simulink model "mcb_pmsm_foc_sensorless_CVAC_IF_f28379d"  (R2026a)
settings: Solver=FixedStepDiscrete  StopTime=8  EnableMultiTasking=on
InitFcn:
  | cvac_if_model_init;
model workspace (MAT data in the model file):
  encoderResolution = 2000
  hallOffset = '0.5'
  indexOffset = 850
  polePairs = '4'
values from neighbouring files (symbols this model uses):
  acceleration = 500 / PU_System.N_base    [cvac_if_model_init.m]
  CVAC_IF_Mode = uint8(2)    [cvac_if_model_init.m]
  CVAC_LoadConstant = CVAC_LoadFinal    [cvac_if_model_init.m]
  PU_System = mcb.getPUSystemParameters(pmsm, inverter)    [cvac_if_model_init.m]
  Speed_openLoop_PU = 400 / PU_System.N_base    [cvac_if_model_init.m]
  Ts = single(param.TsFast)    [cvac_if_reference_fast_step.m]
undefined symbols (not defined in the file or in its folder): bit, CVAC_LoadFinal, CVAC_LoadInitial, CVAC_LoadStepTime, dataType, Down, GPTRIP1SEL, GPTRIP2SEL, inverter, NumBits1, NumBits2, PI_params, pmsm, Slope1, Slope2, target, Ts_motor, Ts_simulink, Ts_speed, TZ1, TZ2, Up
libraries: mcbcontrolslib x9, c2802xlib x7, simulink x6, c280xlib x5, mcbeeMathTransformLib x4, c2837xDlib x4, mcbpositiondecoderlib x3, slpidlib x3, sl_signal_attributes x2, mcbpmsmiflib x2, mcbsensorlessestimatorlib x1, svdschedulerlib x1
(part 1 of 3)
Description:
  | MIL-only CVAC I-f study model using a 540 V paper IPMSM. Do not Build or Deploy.
settings Model: ExtModeTrigDuration=8  Creator=The MathWorks, Inc.  LastModifiedBy=ASUS
settings OptimizationCC: DefaultUnderspecifiedDataType=single  OptimizeBlockIOStorage=off  BufferReuse=off  GlobalBufferReuse=off  ExpressionFolding=off  LocalBlockOutputs=off  InitFltsAndDblsToZero=on  NoFixptDivByZeroProtection=on  EfficientFloat2IntCast=on  EfficientMapNaN2IntZero=off  LifeSpan=Inf  MaxStackSize=1024  OptimizeDataStoreBuffers=off  BusAssignmentInplaceUpdate=off  DenormalBehavior=FlushToZero
settings DebuggingCC: ReadBeforeWriteMsg=DisableAll  WriteAfterWriteMsg=DisableAll  WriteAfterReadMsg=DisableAll  CheckSSInitialOutputMsg=off  InheritedTsInSrcMsg=none  MultiTaskDSMMsg=none  MultiTaskCondExecSysMsg=none  TasksWithSamePriorityMsg=none  SigSpecEnsureSampleTimeMsg=none  IntegerOverflowMsg=none  ParameterPrecisionLossMsg=none  SubsystemReferenceDiagnosticForUnitTest=warning  IntegerSaturationMsg=none
settings HardwareCC: ProdBitPerChar=16.0  ProdBitPerInt=16.0  ProdLargestAtomicInteger=Integer  ProdWordSize=16.0  ProdHWDeviceType=Texas Instruments->C2000  TargetBitPerChar=16.0  TargetBitPerInt=16.0  TargetBitPerPointer=16.0  TargetLargestAtomicInteger=Integer  TargetIntDivRoundTo=Zero  TargetEndianess=LittleEndian  TargetWordSize=16.0  TargetHWDeviceType=TI C2000
settings RTWCC: SystemTargetFile=ert.tlc  HardwareBoard=TI Delfino F28379D LaunchPad  PostCodeGenCommand=error('CVAC_IF_sim:MilOnly', 'MIL-only 540 V paper model: Build and Deploy are intentionally disabled.')  GenerateReport=on  Toolchain=Texas Instruments Code Composer Studio (C2000)  IncludeHyperlinkInReport=on  LaunchReport=on  GenerateTraceInfo=on  GenerateTraceReport=on  GenerateTraceReportSl=on  GenerateTraceReportSf=on  GenerateTraceReportEml=on  Description=Embedded Coder
settings CodeAppCC: CustomSymbolStrType=$N$R$M  InternalIdentifier=Classic
settings ERTTargetCC: ExtModeStaticAllocSize=10000.0  MemSecPackage=tic2000demospkg  CodeReplacementLibrary=TI C28x  MultiwordLength=2048.0
settings SimscapeCC: SimscapeNominalValues="[{\"value\":\"1\",\"unit\":\"A\"},{\"value\":\"1\",\"unit\":\"bar\"},{\"value\":\"1\",\"unit\":\"cm^2\"},{\"value\":\"1\",\"unit\":\"cm^3/s\"},{\"value\":\"1\",\"unit\":\"kJ/kg\"},{\"value\":\"1\",\"unit\":\"kW\"},{\"value\":\"1\",\"unit\":\"l\"},{\"value\":\"1\",\"unit\":\"N\"},{\"value\":\"1\",\"unit\":\"N*m\"},{\"value\":\"1\",\"unit\":\"V\"}]"  SimscapeLogType=none  SimscapeLogDataHistory=5000.0

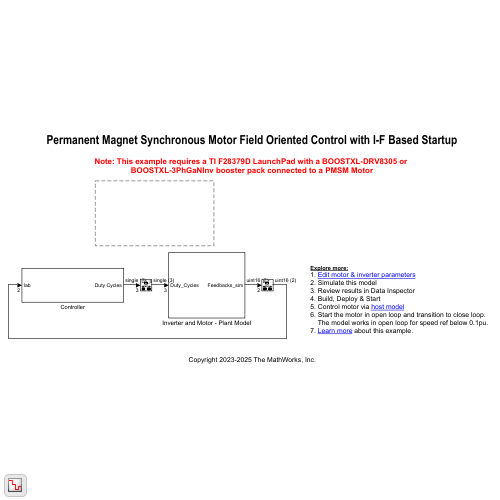
[thumbnail: Simulink's stored preview of the top-level diagram]
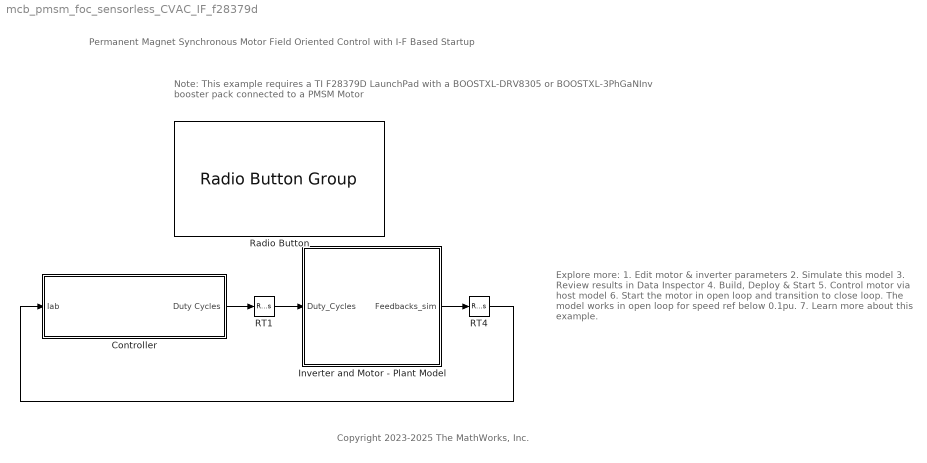
== system mcb_pmsm_foc_sensorless_CVAC_IF_f28379d ==
  note: Permanent Magnet Synchronous Motor Field Oriented Control with I-F Based Startup
  note: Explore more:
      | 1. Edit motor & inverter parameters
      | 2. Simulate this model
      | 3. Review results in Data Inspector
      | 4. Build, Deploy & Start
      | 5. Control motor via host model
      | 6. Start the motor in open loop and transition to close loop.
      | The model works in open loop for speed ref below 0.1pu.
      | 7. Learn more about this example.
  note: Note: This example requires a TI F28379D LaunchPad with a BOOSTXL-DRV8305 or
      | BOOSTXL-3PhGaNInv booster pack connected to a PMSM Motor
  note: Copyright 2023-2025 The MathWorks, Inc.
  Controller : Subsystem
  Inverter and Motor - Plant Model : Subsystem
  RT1 : RateTransition  Deterministic=off
  RT4 : RateTransition  Deterministic=off
  Radio Button : RadioButtonGroup  LabelPosition=Hide  SelectedLabel=Extended Emf observer  ButtonGroupName=Postion Estimator
  wires:
  Inverter and Motor - Plant Model/1(Feedbacks_sim) -> RT4/1
  RT1/1 -> Inverter and Motor - Plant Model/1(Duty_Cycles)
  RT4/1 -> Controller/1(Iab)
  Controller/1(Duty Cycles) -> RT1/1

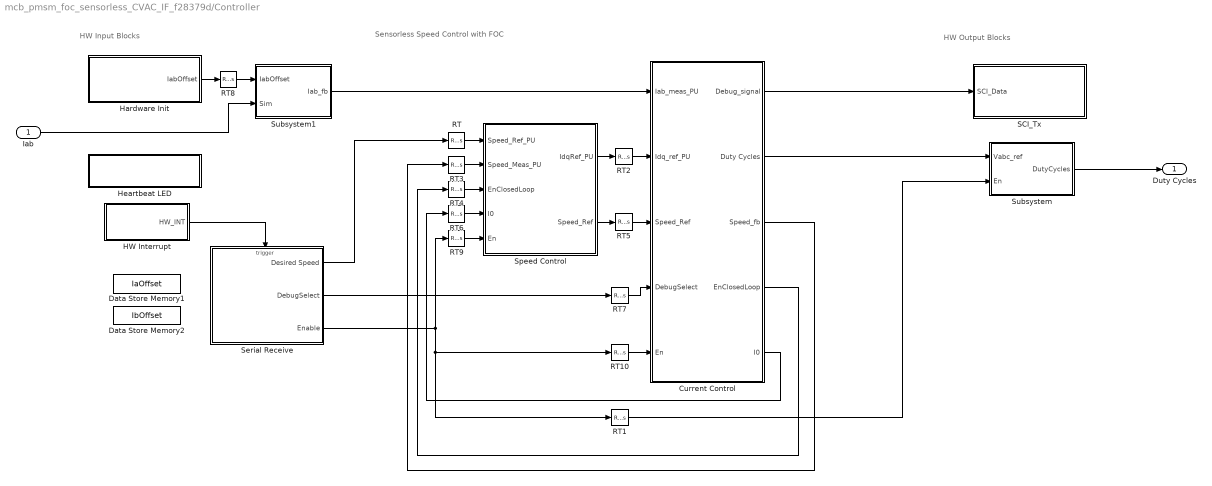
== system mcb_pmsm_foc_sensorless_CVAC_IF_f28379d/Controller ==
  note: HW Input Blocks
  note: Sensorless Speed Control with FOC
  note: HW Output Blocks
  Iab : Inport
  Current Control : Subsystem
  Data Store Memory1 : DataStoreMemory  DataStoreName=IaOffset  InitialValue=inverter.CtSensAOffset  ShowAdditionalParam=off  OutDataTypeStr=uint16
  Data Store Memory2 : DataStoreMemory  DataStoreName=IbOffset  InitialValue=inverter.CtSensBOffset  ShowAdditionalParam=off
  HW Interrupt : Subsystem  Variant=on  VariantControlMode=sim codegen switching
  Hardware Init : Subsystem  TreatAsAtomicUnit=on
  Heartbeat LED : Subsystem  TreatAsAtomicUnit=on
  RT{,3..4,6,9} (5 alike) : RateTransition  Deterministic=off  OutPortSampleTime=Ts_speed
  RT{1..2,5,7..8,10} (6 alike) : RateTransition  Deterministic=off  OutPortSampleTime=Ts
  SCI_Tx : Subsystem  Variant=on  VariantControlMode=sim codegen switching
  Serial Receive : Subsystem  SystemSampleTime=1e-3
  Speed Control : Subsystem  TreatAsAtomicUnit=on  SystemSampleTime=Ts_speed
  Subsystem : Subsystem
  Subsystem1 : Subsystem
  Duty Cycles : Outport
  wires:
  Speed Control/1(IdqRef_PU) -> RT2/1
  RT5/1 -> Current Control/3(Speed_Ref)
  RT/1 -> Speed Control/1(Speed_Ref_PU)
  Current Control/3(Speed_fb) -> RT3/1
  Speed Control/2(Speed_Ref) -> RT5/1
  RT2/1 -> Current Control/2(Idq_ref_PU)
  RT3/1 -> Speed Control/2(Speed_Meas_PU)
  Serial Receive/1(Desired Speed) -> RT/1
  Iab/1 -> Subsystem1/2(Sim)
  HW Interrupt/1(HW_INT) -> Serial Receive/Trigger
  Current Control/1(Debug_signal) -> SCI_Tx/1(SCI_Data)
  Subsystem/1(DutyCycles) -> Duty Cycles/1
  Current Control/2(Duty Cycles) -> Subsystem/1(Vabc_ref)
  Serial Receive/3(Enable) -> RT1/1, RT10/1, RT9/1
  RT10/1 -> Current Control/5(En)
  RT1/1 -> Subsystem/2(En)
  Current Control/4(EnClosedLoop) -> RT4/1
  Current Control/5(I0) -> RT6/1
  RT4/1 -> Speed Control/3(EnClosedLoop)
  RT6/1 -> Speed Control/4(I0)
  Serial Receive/2(DebugSelect) -> RT7/1
  RT7/1 -> Current Control/4(DebugSelect)
  Hardware Init/1(IabOffset) -> RT8/1
  RT8/1 -> Subsystem1/1(IabOffset)
  RT9/1 -> Speed Control/5(En)
  Subsystem1/1(Iab_fb) -> Current Control/1(Iab_meas_PU)

== system mcb_pmsm_foc_sensorless_CVAC_IF_f28379d/Inverter and Motor - Plant Model ==
  Duty_Cycles : Inport
  Codegeneration : Subsystem
  Simulation : Subsystem
  Variant Sink : VariantSink  VariantControlMode=sim codegen switching  VariantControls={(codegen), (sim)}
  Variant Source1 : VariantSource  VariantControlMode=sim codegen switching  VariantControls={(codegen), (sim)}
  Feedbacks_sim : Outport  VectorParamsAs1DForOutWhenUnconnected=off
  wires:
  Duty_Cycles/1 -> Variant Sink/1
  Simulation/1(Feedbacks) -> Variant Source1/2
  Variant Sink/2 -> Simulation/1(Duty_Cycles)
  Variant Source1/1 -> Feedbacks_sim/1
  Variant Sink/1 -> Codegeneration/1(Duty_Cycles)
  Codegeneration/1(Feedbacks) -> Variant Source1/1

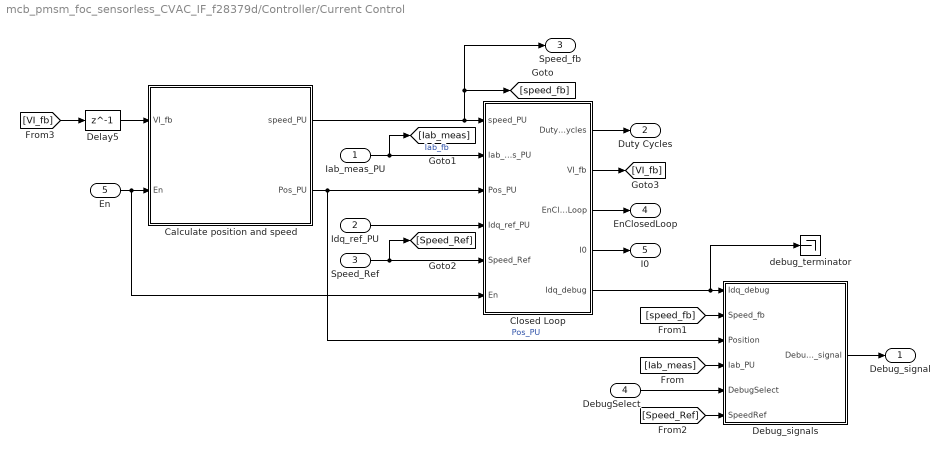
== system mcb_pmsm_foc_sensorless_CVAC_IF_f28379d/Controller/Current Control ==
  Iab_meas_PU : Inport
  Idq_ref_PU : Inport  Port=2
  Speed_Ref : Inport  Port=3
  DebugSelect : Inport  Port=4
  En : Inport  Port=5
  Calculate position and speed : Subsystem
  Closed Loop : Subsystem
  Debug_signals : Subsystem
  Delay5 : Delay  DelayLength=1
  debug_terminator : Terminator
  Debug_signal : Outport
  Duty Cycles : Outport  Port=2  InitialOutput=0  VectorParamsAs1DForOutWhenUnconnected=off
  Speed_fb : Outport  Port=3  InitialOutput=0  VectorParamsAs1DForOutWhenUnconnected=off
  EnClosedLoop : Outport  Port=4
  I0 : Outport  Port=5
  wires:
  Closed Loop/1(Duty Cycles) -> Duty Cycles/1
  Calculate position and speed/2(Pos_PU) -> Closed Loop/3(Pos_PU), Debug_signals/3(Position)  "Pos_PU"
  Idq_ref_PU/1 -> Closed Loop/4(Idq_ref_PU)
  Iab_meas_PU/1 -> Closed Loop/2(Iab_meas_PU), [Iab_meas]  "Iab_fb"
  Closed Loop/2(VI_fb) -> [VI_fb]
  [VI_fb] -> Delay5/1
  Calculate position and speed/1(speed_PU) -> Closed Loop/1(speed_PU), [speed_fb], Speed_fb/1
  Closed Loop/5(Idq_debug) -> debug_terminator/1, Debug_signals/1(Idq_debug)
  [speed_fb] -> Debug_signals/2(Speed_fb)
  Debug_signals/1(Debug_signal) -> Debug_signal/1
  Delay5/1 -> Calculate position and speed/1(VI_fb)
  En/1 -> Closed Loop/6(En), Calculate position and speed/2(En)
  DebugSelect/1 -> Debug_signals/5(DebugSelect)
  Speed_Ref/1 -> Closed Loop/5(Speed_Ref), [Speed_Ref]
  Closed Loop/3(EnClosedLoop) -> EnClosedLoop/1
  Closed Loop/4(I0) -> I0/1
  [Iab_meas] -> Debug_signals/4(Iab_PU)
  [Speed_Ref] -> Debug_signals/6(SpeedRef)

== system mcb_pmsm_foc_sensorless_CVAC_IF_f28379d/Controller/HW Interrupt ==
  Code generation : Subsystem  VariantControl=(codegen)
  Simulation : Subsystem  VariantControl=(sim)
  HW_INT : Outport  OutputFunctionCall=on

== system mcb_pmsm_foc_sensorless_CVAC_IF_f28379d/Controller/Hardware Init ==
  6PWM_Mode : Constant  Priority=1000  Value=0x3A16  OutDataTypeStr=uint16  SampleTime=-1
  ADC_Gain_Setting : Constant  Priority=1000  Value=inverter.SPI_Gain_Setting  OutDataTypeStr=uint16  SampleTime=-1
  Data Store Read1 : DataStoreRead  DataStoreName=IaOffset  IndexOptions=Index vector (dialog)  Indices=1  OutputSizes=1
  Data Store Read2 : DataStoreRead  DataStoreName=IbOffset  IndexOptions=Index vector (dialog)  Indices=1  OutputSizes=1
  Event Listener : EventListener  DisableCoverage=on  EventName=reset
  Mux : Mux  Inputs=2
  Mux1 : Mux  Inputs=2
  Variant Subsystem : Subsystem  Variant=on  VariantControlMode=sim codegen switching
  IabOffset : Outport
  wires:
  6PWM_Mode/1 -> Mux/1
  ADC_Gain_Setting/1 -> Mux/2
  Mux/1 -> Variant Subsystem/1(In1)
  Mux1/1 -> IabOffset/1
  Data Store Read1/1 -> Mux1/1
  Data Store Read2/1 -> Mux1/2

== system mcb_pmsm_foc_sensorless_CVAC_IF_f28379d/Controller/Heartbeat LED ==
  note: Heartbeat LED 1 Hz
  Heartbeat LED : Subsystem  Variant=on  VariantControlMode=sim codegen switching
  RED_LED : Constant  OutDataTypeStr=uint16  SampleTime=0.5
  wires:
  RED_LED/1 -> Heartbeat LED/1(In1)

== system mcb_pmsm_foc_sensorless_CVAC_IF_f28379d/Controller/SCI_Tx ==
  SCI_Data : Inport
  Code Generation : Subsystem  VariantControl=(codegen)
  Simulation : Subsystem  VariantControl=(sim)

== system mcb_pmsm_foc_sensorless_CVAC_IF_f28379d/Controller/Serial Receive ==
  SCI_Rx_INT : TriggerPort  TriggerType=function-call  VariantControl=Variant
  AND : Logic  IconShape=distinctive  AllPortsSameDT=off  OutDataTypeStr=boolean
  Compare To Zero : simulink/Logic and Bit Operations/Compare To Zero  relop=~=  OutDataTypeStr=boolean
  Data_Conditioning_Rx : Subsystem  Variant=on
  SCI_Rx : Subsystem  Variant=on  VariantControlMode=sim codegen switching
  unParse : Subsystem
  Desired Speed : Outport  VectorParamsAs1DForOutWhenUnconnected=off
  DebugSelect : Outport  Port=2
  Enable : Outport  Port=3  VectorParamsAs1DForOutWhenUnconnected=off
  wires:
  unParse/2(Debug_signals) -> DebugSelect/1
  unParse/1(Enable_PWM) -> AND/2
  Data_Conditioning_Rx/2(Out2) -> unParse/1(Data)
  SCI_Rx/1(Data) -> Data_Conditioning_Rx/1(In1)
  Data_Conditioning_Rx/1(Desired Speed) -> Compare To Zero/1, Desired Speed/1
  Compare To Zero/1 -> AND/1
  AND/1 -> Enable/1

== system mcb_pmsm_foc_sensorless_CVAC_IF_f28379d/Controller/Speed Control ==
  Speed_Ref_PU : Inport
  Speed_Meas_PU : Inport  Port=2
  EnClosedLoop : Inport  Port=3
  I0 : Inport  Port=4
  En : Inport  Port=5
  Constant2 : Constant  Value=0  OutDataTypeStr=dataType
  Mux : Mux  Inputs=2
  PI_Controller_Speed : Subsystem
  SlewRate1 : Subsystem
  Switch : Switch  Criteria=u2 > Threshold  SaturateOnIntegerOverflow=off  InputSameDT=off
  IdqRef_PU : Outport  VectorParamsAs1DForOutWhenUnconnected=off
  Speed_Ref : Outport  Port=2  VectorParamsAs1DForOutWhenUnconnected=off
  wires:
  Speed_Meas_PU/1 -> PI_Controller_Speed/2(N_fb)  "Speed_fb"
  Mux/1 -> IdqRef_PU/1
  Constant2/1 -> Mux/1
  PI_Controller_Speed/1(Iq_ref) -> Mux/2
  Switch/1 -> Speed_Ref/1, PI_Controller_Speed/1(N_ref)
  EnClosedLoop/1 -> PI_Controller_Speed/3(EnClosedLoop), Switch/2, SlewRate1/2(EnClosedLoop)
  SlewRate1/1(N_ref) -> Switch/1  "Speed_ref"
  Speed_Ref_PU/1 -> SlewRate1/1(Speed_Ref), Switch/3  "Speed_ref"
  I0/1 -> PI_Controller_Speed/4(I0)
  En/1 -> PI_Controller_Speed/5(En)

== system mcb_pmsm_foc_sensorless_CVAC_IF_f28379d/Controller/Subsystem ==
  Vabc_ref : Inport
  En : Inport  Port=2
  Inverter : Subsystem  Variant=on  VariantControlMode=sim codegen switching
  Mux : Mux  Inputs=2
  Output Scaling : Subsystem
  DutyCycles : Outport
  wires:
  Output Scaling/1(PWM_Duty_Cycles) -> Mux/1
  Mux/1 -> Inverter/1(Inverter Signals)
  Output Scaling/2(PWM_Enable) -> Mux/2
  Inverter/1(DutyCycles) -> DutyCycles/1
  En/1 -> Output Scaling/2(En)
  Vabc_ref/1 -> Output Scaling/1(Vabc_ref)

== system mcb_pmsm_foc_sensorless_CVAC_IF_f28379d/Controller/Subsystem1 ==
  IabOffset : Inport
  Sim : Inport  Port=2
  Calculate Phase Currents : Subsystem
  HW_Inputs : Subsystem  Variant=on  VariantControlMode=sim codegen switching
  Iab_fb : Outport
  wires:
  HW_Inputs/1(Iab_ADC) -> Calculate Phase Currents/2(Iab_ADC)
  IabOffset/1 -> Calculate Phase Currents/1(IabOffset)
  Calculate Phase Currents/1(Iab_meas_PU) -> Iab_fb/1  "Iab_fb"
  Sim/1 -> HW_Inputs/1(Sim)

== system mcb_pmsm_foc_sensorless_CVAC_IF_f28379d/Inverter and Motor - Plant Model/Codegeneration ==
  Duty_Cycles : Inport
  Ground : Ground
  Terminator : Terminator
  Feedbacks : Outport  VectorParamsAs1DForOutWhenUnconnected=off
  wires:
  Duty_Cycles/1 -> Terminator/1
  Ground/1 -> Feedbacks/1

== system mcb_pmsm_foc_sensorless_CVAC_IF_f28379d/Inverter and Motor - Plant Model/Simulation ==
  Duty_Cycles : Inport
  Bus Selector : BusSelector  OutputSignals=MtrPos
  Gain : Gain  Gain=1/(2*pi)  OutDataTypeStr=Inherit: Same as input
  Interior_PMSM_Paper : autolibpmsminterior/Interior PMSM  port_config=Torque  sim_type=Discrete  Ts=Ts_motor  P=pmsm.p  Rs=pmsm.Rs  Ldq=[pmsm.Ld,pmsm.Lq]  KConstText=Permanent flux linkage constant (lambda_pm):  lambda_pm=pmsm.FluxPM  Ke=159.9771  mechanical=[pmsm.J,pmsm.B,0]  idq0=[0 0]  theta_init=0  omega_init=0  KConst=pmsm.FluxPM  lambda_pm_calc=0.2205  Kt=0.07  RefBlkName='autolibpmsminterior/Interior PMSM'  aMode=1
  Inverter : Subsystem
  Load_Profile (Torque) : Subsystem
  Mechanical to Electrical Position : mcbpositiondecoderlib/Mechanical to Electrical Position  PolePairsInputType=Specify via dialog  NrPP=pmsm.p  selectedRange=Radians  MechOfstInputType=Specify via dialog  mechOffsetIn=0  maxAngleIn=2*pi  InputDataType=single  VariantSelect=floating-point
  RT1 : RateTransition  Deterministic=off  OutPortSampleTime=Ts_simulink
  Rate Transition : RateTransition  Deterministic=off  OutPortSampleTime=Ts_motor
  Rate Transition1 : RateTransition  Deterministic=off  OutPortSampleTime=Ts_motor
  Sensor_Measurements : Subsystem
  Terminator : Terminator
  Terminator1 : Terminator
  Feedbacks : Outport  VectorParamsAs1DForOutWhenUnconnected=off
  wires:
  Mechanical to Electrical Position/1 -> Gain/1  "MtrPosElec"
  Duty_Cycles/1 -> Inverter/1(Duty_abc)
  RT1/1 -> Sensor_Measurements/1(PhaseCurr)
  Load_Profile (Torque)/1(Load_Trq) -> Rate Transition1/1
  Inverter/1(Vabc) -> Rate Transition/1
  Bus Selector/1 -> Mechanical to Electrical Position/1  "<MtrPos>"
  Gain/1 -> Terminator1/1  "MtrPosElec"
  Sensor_Measurements/1(Sim_fb) -> Feedbacks/1
  Rate Transition1/1 -> Interior_PMSM_Paper/1
  Rate Transition/1 -> Interior_PMSM_Paper/2
  Interior_PMSM_Paper/1 -> Bus Selector/1
  Interior_PMSM_Paper/2 -> RT1/1  "Iabc"
  Interior_PMSM_Paper/3 -> Terminator/1  "MtrSpdTrue"

== system mcb_pmsm_foc_sensorless_CVAC_IF_f28379d/Controller/Current Control/Calculate position and speed ==
  VI_fb : Inport
  En : Inport  Port=2
  Demux : Demux  Outputs=2
  EstimatorSelector : Constant  OutDataTypeStr=uint32
  Extended EMF Observer : Subsystem
  Flux Observer : Subsystem
  Merge : Merge
  Switch Case : SwitchCase  CaseConditions={0,1}  ShowDefaultCase=off
  speed_PU : Outport
  Pos_PU : Outport  Port=2
  wires:
  Demux/1 -> Pos_PU/1
  Demux/2 -> speed_PU/1
  EstimatorSelector/1 -> Switch Case/1
  Flux Observer/1(Position/Speed) -> Merge/1
  Merge/1 -> Demux/1
  VI_fb/1 -> Extended EMF Observer/1(InputSignals), Flux Observer/1(InputSignals)
  Extended EMF Observer/1(Position/Speed) -> Merge/2
  Switch Case/2 -> Extended EMF Observer/Action
  Switch Case/1 -> Flux Observer/Action
  En/1 -> Extended EMF Observer/2(En), Flux Observer/2(En)

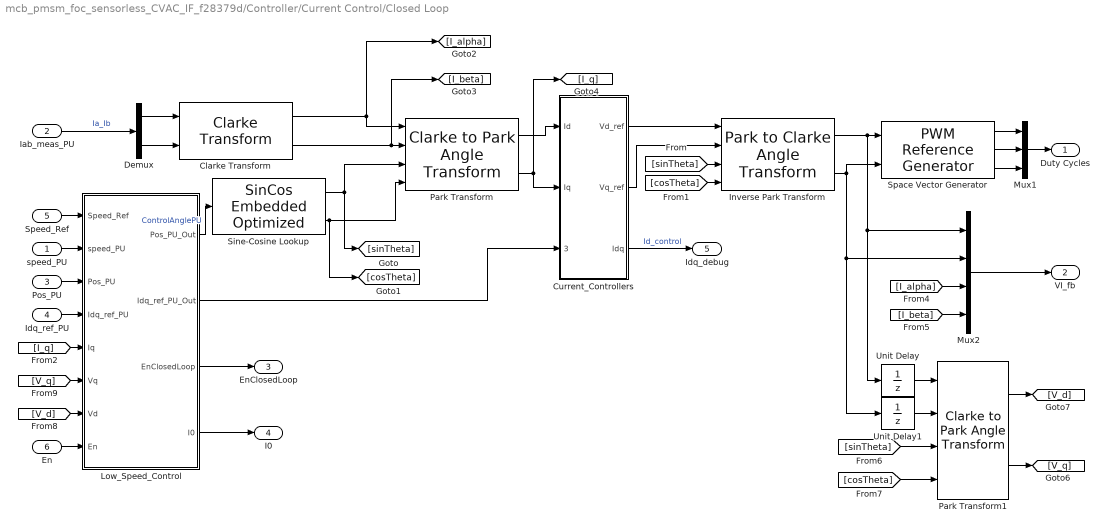
== system mcb_pmsm_foc_sensorless_CVAC_IF_f28379d/Controller/Current Control/Closed Loop ==
  speed_PU : Inport
  Iab_meas_PU : Inport  Port=2
  Pos_PU : Inport  Port=3
  Idq_ref_PU : Inport  Port=4
  Speed_Ref : Inport  Port=5
  En : Inport  Port=6
  Clarke Transform : mcbeeMathTransformLib/Clarke Transform  VariantControl=Variant2  PowerInvariant=off  UseWithEmbedded=on  PhaseInput=Two inputs
      settings: LibrarySourceBlock=mcbcontrolslib/Clarke Transform
  Current_Controllers : Subsystem
  Demux : Demux  Outputs=2
  Inverse Park Transform : mcbeeMathTransformLib/Park to Clarke Angle Transform  AxisAlignment=D-axis  UseWithEmbedded=on  PhaseInput=Two inputs  ThetaInput=Sine and Cosine electrical position  AngleInput=Per-unit  N_points=1024
      settings: LibrarySourceBlock=mcbcontrolslib/Inverse Park Transform
  Low_Speed_Control : Subsystem
  Mux1 : Mux  Inputs=3
  Mux2 : Mux
  Park Transform : mcbeeMathTransformLib/Clarke to Park Angle Transform  AxisAlignment=D-axis  UseWithEmbedded=on  PhaseInput=Two inputs  ThetaInput=Sine and Cosine electrical position  AngleInput=Per-unit  N_points=1024
      settings: LibrarySourceBlock=mcbcontrolslib/Park Transform
  Park Transform1 : mcbeeMathTransformLib/Clarke to Park Angle Transform  AxisAlignment=D-axis  UseWithEmbedded=on  PhaseInput=Two inputs  ThetaInput=Sine and Cosine electrical position  AngleInput=Per-unit  N_points=1024
      settings: LibrarySourceBlock=mcbcontrolslib/Park Transform
  Sine-Cosine Lookup : mcbcontrolslib/SinCos Embedded Optimized  LabelModeActiveChoice=MCB_Sin  OptforProc=off  OptLevelPop=Disabled  ApproximationMethod=None  UserApproxMethod=Lookup  ApproxStatus=None  ThetaDataType=single  CopyThetaDataType=single  InterpMethod=Linear point-slope  NumberOfDataPoints=16  NumberOfIterations=11  RemoveProtectionAgainstOutOfRangeInput=off  TableDataTypeStr=Inherit: Inherit via input  AngleInput=Per-unit  CopyAngleInput=Per-unit  N_points=1024  CopyN_points=1024  Datatype=single  CopyTableDatatype=single  DatatypeInput=Inherit from input  IsPrevStrictOpt=0  IsPrevLUTForced=0
  Space Vector Generator : mcbcontrolslib/PWM Reference Generator  modType=SVM: space vector modulation  inSignal=Valphabeta  expandVoltageInput=on  inputUnits=Per-unit  LimitModulation=off  enableVoltage=on  enableModulationSignal=off  enableDutyCycle=off  expandVoltageOutput=on
  Unit Delay : UnitDelay  SampleTime=-1
  Unit Delay1 : UnitDelay  SampleTime=-1
  Duty Cycles : Outport  VectorParamsAs1DForOutWhenUnconnected=off
  VI_fb : Outport  Port=2  VectorParamsAs1DForOutWhenUnconnected=off
  EnClosedLoop : Outport  Port=3
  I0 : Outport  Port=4
  Idq_debug : Outport  Port=5  VectorParamsAs1DForOutWhenUnconnected=off
  wires:
  Current_Controllers/1(Vd_ref) -> Inverse Park Transform/1
  [cosTheta] -> Inverse Park Transform/4
  [I_beta] -> Mux2/4
  Inverse Park Transform/2 -> Mux2/2, Unit Delay1/1, Space Vector Generator/2
  Inverse Park Transform/1 -> Mux2/1, Unit Delay/1, Space Vector Generator/1
  [sinTheta] -> Inverse Park Transform/3
  Mux2/1 -> VI_fb/1
  Clarke Transform/1 -> Park Transform/1, [I_alpha]
  Current_Controllers/2(Vq_ref) -> Inverse Park Transform/2
  Clarke Transform/2 -> [I_beta], Park Transform/2
  Sine-Cosine Lookup/1 -> Park Transform/3, [sinTheta]
  [I_alpha] -> Mux2/3
  Space Vector Generator/1 -> Mux1/1
  Space Vector Generator/3 -> Mux1/3
  Mux1/1 -> Duty Cycles/1
  Sine-Cosine Lookup/2 -> Park Transform/4, [cosTheta]
  Space Vector Generator/2 -> Mux1/2
  Park Transform/1 -> Current_Controllers/1(Id)
  Park Transform/2 -> Current_Controllers/2(Iq), [I_q]
  Demux/1 -> Clarke Transform/1
  Demux/2 -> Clarke Transform/2
  Iab_meas_PU/1 -> Demux/1  "Ia_Ib"
  Pos_PU/1 -> Low_Speed_Control/3(Pos_PU)
  Current_Controllers/3(Idq) -> Idq_debug/1  "Id_control"
  Low_Speed_Control/1(Pos_PU_Out) -> Sine-Cosine Lookup/1  "ControlAnglePU"
  speed_PU/1 -> Low_Speed_Control/2(speed_PU)
  Idq_ref_PU/1 -> Low_Speed_Control/4(Idq_ref_PU)
  [I_q] -> Low_Speed_Control/5(Iq)
  Low_Speed_Control/2(Idq_ref_PU_Out) -> Current_Controllers/3(Idq_Ref)
  Speed_Ref/1 -> Low_Speed_Control/1(Speed_Ref)
  Unit Delay/1 -> Park Transform1/1
  Unit Delay1/1 -> Park Transform1/2
  [sinTheta] -> Park Transform1/3
  [cosTheta] -> Park Transform1/4
  Park Transform1/1 -> [V_d]
  Park Transform1/2 -> [V_q]
  [V_d] -> Low_Speed_Control/7(Vd)
  [V_q] -> Low_Speed_Control/6(Vq)
  En/1 -> Low_Speed_Control/8(En)
  Low_Speed_Control/3(EnClosedLoop) -> EnClosedLoop/1
  Low_Speed_Control/4(I0) -> I0/1

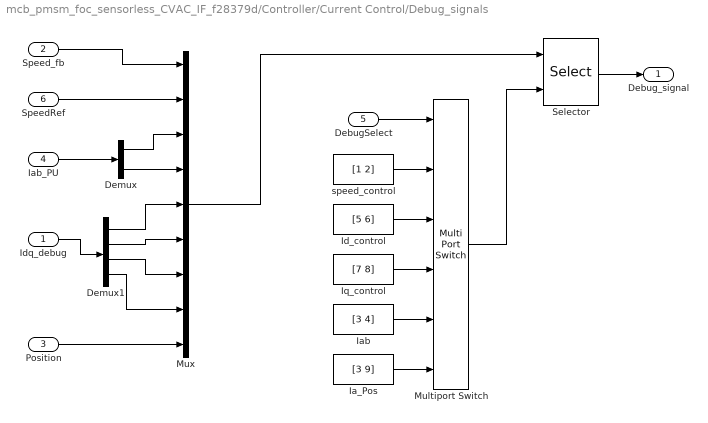
== system mcb_pmsm_foc_sensorless_CVAC_IF_f28379d/Controller/Current Control/Debug_signals ==
  Idq_debug : Inport
  Speed_fb : Inport  Port=2
  Position : Inport  Port=3
  Iab_PU : Inport  Port=4
  DebugSelect : Inport  Port=5
  SpeedRef : Inport  Port=6
  Demux : Demux  Outputs=2
  Demux1 : Demux
  Ia_Pos : Constant  Value=[3 9]  OutDataTypeStr=uint16  SampleTime=-1
  Iab : Constant  Value=[3 4]  OutDataTypeStr=uint16  SampleTime=-1
  Id_control : Constant  Value=[5 6]  OutDataTypeStr=uint16  SampleTime=-1
  Iq_control : Constant  Value=[7 8]  OutDataTypeStr=uint16  SampleTime=-1
  Multiport Switch : MultiPortSwitch  Inputs=5  DiagnosticForDefault=Warning  OutDataTypeStr=uint16  RndMeth=Simplest  SaturateOnIntegerOverflow=off  InputSameDT=off
  Mux : Mux  Inputs=9
  Selector : Selector  InputPortWidth=9  IndexOptions=Index vector (port)  Indices=[1 3]  OutputSizes=1
  speed_control : Constant  Value=[1 2]  OutDataTypeStr=uint16  SampleTime=-1
  Debug_signal : Outport
  wires:
  speed_control/1 -> Multiport Switch/2
  Id_control/1 -> Multiport Switch/3
  Iq_control/1 -> Multiport Switch/4
  Iab/1 -> Multiport Switch/5
  Ia_Pos/1 -> Multiport Switch/6
  Multiport Switch/1 -> Selector/2
  DebugSelect/1 -> Multiport Switch/1
  Selector/1 -> Debug_signal/1
  SpeedRef/1 -> Mux/2
  Iab_PU/1 -> Demux/1
  Demux/1 -> Mux/3
  Demux/2 -> Mux/4
  Demux1/1 -> Mux/5
  Demux1/2 -> Mux/6
  Demux1/3 -> Mux/7
  Demux1/4 -> Mux/8
  Idq_debug/1 -> Demux1/1
  Mux/1 -> Selector/1
  Speed_fb/1 -> Mux/1
  Position/1 -> Mux/9

== system mcb_pmsm_foc_sensorless_CVAC_IF_f28379d/Controller/HW Interrupt/Code generation ==
  HWI_SCIA_RX_INT : svdschedulerlib/Hardware Interrupt v2  ISRGroup=ADC - Analog to Digital Converter  ISRName=ADCA1_INT  ISRNumber=32  NumEventsToServe=1  EventsList={'on','EOC event','1';'off','Overflow event','2';'off','Custom event','3'}  SelectedEvents={'event1'}  TaskPriority=50  DisablePreemption=on  ClearInterruptFlagsAtEndOfEvent=on  InterruptDefinitionFile=$(TARGET_ROOT)/registry/interrupts/F2837xS_interrupts.xml  HardwareBoard=F2837x  EnableSimPort=off
      settings: LibrarySourceBlock=c2000lib/Scheduling/Hardware Interrupt
  HW_INT : Outport
  wires:
  HWI_SCIA_RX_INT/1 -> HW_INT/1

== system mcb_pmsm_foc_sensorless_CVAC_IF_f28379d/Controller/HW Interrupt/Simulation ==
  SCI_Rx_INT : FunctionCallGenerator  SampleTime=0.1
  HW_INT : Outport
  wires:
  SCI_Rx_INT/1 -> HW_INT/1

== system mcb_pmsm_foc_sensorless_CVAC_IF_f28379d/Controller/Hardware Init/Variant Subsystem ==
  In1 : Inport
  Code Generation : Subsystem  VariantControl=(codegen)
  Simulation : Subsystem  VariantControl=(sim)

== system mcb_pmsm_foc_sensorless_CVAC_IF_f28379d/Controller/Heartbeat LED/Heartbeat LED ==
  In1 : Inport
  Code generation : Subsystem  VariantControl=(codegen)
  Simulation : Subsystem  VariantControl=(sim)

== system mcb_pmsm_foc_sensorless_CVAC_IF_f28379d/Controller/SCI_Tx/Code Generation ==
  SCI_Data : Inport
  Data_Conditioning_Tx : Subsystem  Variant=on
  Data_Logging : Subsystem
  Demux2 : Demux  Outputs=2
  While Iterator Subsystem : Subsystem  TreatAsAtomicUnit=on
  wires:
  Demux2/2 -> While Iterator Subsystem/2(Iteration)  "SCI_Tx_Iteration"
  Demux2/1 -> While Iterator Subsystem/1(Data)  "SCI_Tx_Data"
  SCI_Data/1 -> Data_Conditioning_Tx/1(In1)
  Data_Logging/1(SCI_Tx) -> Demux2/1
  Data_Conditioning_Tx/1(Data_Log) -> Data_Logging/1(Data_Log)

== system mcb_pmsm_foc_sensorless_CVAC_IF_f28379d/Controller/SCI_Tx/Simulation ==
  SCI_Data : Inport
  Demux : Demux  Outputs=2
  Terminator1 : Terminator
  Terminator2 : Terminator
  wires:
  SCI_Data/1 -> Demux/1
  Demux/1 -> Terminator1/1
  Demux/2 -> Terminator2/1

== system mcb_pmsm_foc_sensorless_CVAC_IF_f28379d/Controller/Serial Receive/Data_Conditioning_Rx ==
  In1 : Inport
  Data_Type_Fixed_Point : Subsystem  VariantControl=~isequal(dataType, 'single')
  Data_Type_Float : Subsystem  VariantControl=isequal(dataType, 'single')
  Desired Speed : Outport
  Out2 : Outport  Port=2

== system mcb_pmsm_foc_sensorless_CVAC_IF_f28379d/Controller/Serial Receive/SCI_Rx ==
  Code Generation : Subsystem  Variant=on  VariantControl=(codegen)
  Simulation : Subsystem  VariantControl=(sim)
  Data : Outport

== system mcb_pmsm_foc_sensorless_CVAC_IF_f28379d/Controller/Serial Receive/unParse ==
  Data : Inport
  Bitwise Operator : simulink/Logic and Bit Operations/Bitwise Operator  logicop=AND  UseBitMask=on  BitMask=hex2dec('0001')  BitMaskRealWorld=Stored Integer
  Bitwise Operator1 : simulink/Logic and Bit Operations/Bitwise Operator  logicop=AND  UseBitMask=on  BitMask=hex2dec('00F0')  BitMaskRealWorld=Stored Integer
  Data Type Conversion3 : DataTypeConversion  OutDataTypeStr=boolean  RndMeth=Simplest  SaturateOnIntegerOverflow=off
  Data Type Conversion4 : DataTypeConversion  OutDataTypeStr=uint16  RndMeth=Simplest  SaturateOnIntegerOverflow=off
  Shift Arithmetic1 : ArithShift  BitShiftNumber=4
  Enable_PWM : Outport
  Debug_signals : Outport  Port=2
  wires:
  Bitwise Operator1/1 -> Shift Arithmetic1/1
  Data/1 -> Bitwise Operator/1, Bitwise Operator1/1
  Bitwise Operator/1 -> Data Type Conversion3/1
  Data Type Conversion4/1 -> Debug_signals/1
  Shift Arithmetic1/1 -> Data Type Conversion4/1
  Data Type Conversion3/1 -> Enable_PWM/1

== system mcb_pmsm_foc_sensorless_CVAC_IF_f28379d/Controller/Speed Control/PI_Controller_Speed ==
  N_ref : Inport
  N_fb : Inport  Port=2
  EnClosedLoop : Inport  Port=3
  I0 : Inport  Port=4
  En : Inport  Port=5
  AND : Logic  IconShape=distinctive  AllPortsSameDT=off  OutDataTypeStr=boolean
  Discrete PI Controller with anti-windup & reset : slpidlib/PID Controller  Controller=PI  Form=Parallel  TimeDomain=Discrete-time  UseExternalTs=off  SampleTime=-1  IntegratorMethod=Forward Euler  FilterMethod=Forward Euler  ControllerParametersSource=external  P=1  I=1  UseKiTs=on  D=0  UseExternalDerivativeSource=off  N=100  UseFilter=on  TunerSelectOption=Transfer Function Based (PID Tuner App)  InitialConditionSource=external  InitialConditionForIntegrator=0  InitialConditionForFilter=0  DifferentiatorICPrevScaledInput=0  ExternalReset=level  TrackingMode=off  Kt=1  LimitOutput=on  SatLimitsSource=internal  UpperSaturationLimit=1  LowerSaturationLimit=-1  LinearizeAsGain=on  AntiWindupMode=clamping  Kb=1  LimitIntegrator=off  UpperIntegratorSaturationLimit=inf  LowerIntegratorSaturationLimit=-inf  RndMeth=Simplest  POutMin=[]  POutMax=[]  IOutMin=[]  IOutMax=[]  DOutMin=[]  DOutMax=[]  NOutMin=[]  NOutMax=[]  SumOutMin=[]  SumOutMax=[]  SaturationOutDataTypeStr=Inherit: Inherit via back propagation  SaturationOutMin=[]  SaturationOutMax=[]  PParamMin=[]  PParamMax=[]  IParamMin=[]  IParamMax=[]  DParamMin=[]  DParamMax=[]  NParamMin=[]  NParamMax=[]  KbParamMin=[]  KbParamMax=[]  KtParamMin=[]  KtParamMax=[]  KbOutMin=[]  KbOutMax=[]  KtOutMin=[]  KtOutMax=[]  IntegratorOutMin=[]  IntegratorOutMax=[]  FilterOutMin=[]  FilterOutMax=[]  SumI1OutMin=[]  SumI1OutMax=[]  SumI2OutMin=[]  SumI2OutMax=[]  SumI3OutMin=[]  SumI3OutMax=[]  SumI4OutMin=[]  SumI4OutMax=[]  SumDOutMin=[]  SumDOutMax=[]  DifferentiatorOutMin=[]  DifferentiatorOutMax=[]  FilterDiffOutCoefMin=[]  FilterDiffOutCoefMax=[]  ReciprocalOutMin=[]  ReciprocalOutMax=[]  SumDenOutMin=[]  SumDenOutMax=[]  SumNumOutMin=[]  SumNumOutMax=[]  DivideOutMin=[]  DivideOutMax=[]  UdiffTsProdOutMin=[]  UdiffTsProdOutMax=[]  NTsProdOutMin=[]  NTsProdOutMax=[]  UintegralTsProdOutMin=[]  UintegralTsProdOutMax=[]  UngainTsProdOutMin=[]  UngainTsProdOutMax=[]  ClampingZeroOutDataTypeStr=Inherit: Inherit via back propagation  ClampingZeroOutMin=[]  ClampingZeroOutMax=[]  FilterDenConstantOutDataTypeStr=Inherit: Inherit via back propagation  FilterDenConstantOutMin=[]  FilterDenConstantOutMax=[]  PCopyOutDataTypeStr=Inherit: Inherit via back propagation  PCopyOutMin=[]  PCopyOutMax=[]  NCopyOutDataTypeStr=Inherit: Inherit via back propagation  NCopyOutMin=[]  NCopyOutMax=[]  IntegratorContinuousStateAttributes=''  IntegratorStateMustResolveToSignalObject=off  IntegratorRTWStateStorageClass=Auto  FilterContinuousStateAttributes=''  FilterStateMustResolveToSignalObject=off  FilterRTWStateStorageClass=Auto  ParallelPVariant=ExternalParameters  IdealPVariant=Disabled  IVariant=ExternalParameters  DVariant=Disabled  IntegratorVariant=Discrete  SatVariant=Enabled  AWVariant=DiscClampingParallel  PCopyVariant=Disabled  TRVariant=Disabled  FdbkBlocksVariant=Forward  IdealPFdbkVariant=Disabled  SatFdbkVariant=Disabled  DerivativeFilterVariant=Disabled  NVariant=Disabled  NCopyVariant=Disabled_SignalSpec  FilterICVariant=Disabled  IntegratorICVariant=ExternalICs  ExternalResetVariant=ExternalReset  TRSumVariant=Passthrough  SumFdbkVariant=Disabled  SumVariant=Sum_PI  TsampFilterVariant=InternalTs  TsampNgainVariant=Passthrough  TsampIntegralVariant=Disabled_SignalSpec  ExternalSaturationOutDataTypeStr=Inherit: Same as second input  DerivativeSourceVariant=Disabled  PreIntVariant=InternalPreInt
      settings: LibrarySourceBlock=mcbcontrolslib/PI Controller
  Ki1 : Constant  Value=PI_params.Ki_speed*Ts_speed  OutDataTypeStr=dataType  SampleTime=-1
  Kp1 : Constant  Value=PI_params.Kp_speed  OutDataTypeStr=dataType  SampleTime=-1
  Logical Operator : Logic  Operator=NOT  IconShape=distinctive  AllPortsSameDT=off  OutDataTypeStr=boolean
  Sum : Sum  Inputs=|+-  OutDataTypeStr=Inherit: Same as first input
  Switch : Switch  Criteria=u2 > Threshold  SaturateOnIntegerOverflow=off  InputSameDT=off
  Zero_Cancellation : mcbcontrolslib/IIR Filter  VariantControl=Low Pass Filter  VariantSelect=Low-pass  FilterConstantInputType=Specify via dialog  Filter_constant=0.01*(Ts_speed/Ts)  InitialOutput=Specify via dialog  InitialOutputValue=0  ExternalReset=none  advancedSettings=off  Ts=50e-6  cutOff_freq=353.6777
  Iq_ref : Outport  VectorParamsAs1DForOutWhenUnconnected=off
  wires:
  Discrete PI Controller with anti-windup & reset/1 -> Iq_ref/1
  Ki1/1 -> Discrete PI Controller with anti-windup & reset/3
  Kp1/1 -> Discrete PI Controller with anti-windup & reset/2
  N_ref/1 -> Switch/1
  Sum/1 -> Discrete PI Controller with anti-windup & reset/1
  Logical Operator/1 -> Discrete PI Controller with anti-windup & reset/4
  I0/1 -> Discrete PI Controller with anti-windup & reset/5
  En/1 -> AND/1
  AND/1 -> Logical Operator/1
  Zero_Cancellation/1 -> Sum/1
  EnClosedLoop/1 -> AND/2, Switch/2
  N_fb/1 -> Sum/2, Switch/3
  Switch/1 -> Zero_Cancellation/1

== system mcb_pmsm_foc_sensorless_CVAC_IF_f28379d/Controller/Speed Control/SlewRate1 ==
  Speed_Ref : Inport
  EnClosedLoop : Inport  Port=2
  Constant : Constant  Value=Speed_openLoop_PU  OutDataTypeStr=Inherit: Inherit via back propagation  SampleTime=-1
  Constant1 : Constant  Value=-Speed_openLoop_PU  OutDataTypeStr=Inherit: Inherit via back propagation  SampleTime=-1
  Rate Limiter : RateLimiter  RisingSlewLimit=acceleration  FallingSlewLimit=-acceleration  SampleTimeMode=inherited  InitialCondition=Speed_openLoop_PU
  Rate Limiter1 : RateLimiter  RisingSlewLimit=acceleration  FallingSlewLimit=-acceleration  SampleTimeMode=inherited  InitialCondition=-Speed_openLoop_PU
  Switch : Switch  SaturateOnIntegerOverflow=off  InputSameDT=off
  Switch1 : Switch  SaturateOnIntegerOverflow=off  InputSameDT=off
  Switch2 : Switch  Criteria=u2 > Threshold  SaturateOnIntegerOverflow=off  InputSameDT=off
  N_ref : Outport
  wires:
  Rate Limiter/1 -> Switch/1
  Rate Limiter1/1 -> Switch/3
  Speed_Ref/1 -> Switch1/2, Switch2/1
  Switch/1 -> N_ref/1
  Constant/1 -> Switch1/1
  Constant1/1 -> Switch1/3
  EnClosedLoop/1 -> Switch2/2
  Switch1/1 -> Switch2/3
  Switch2/1 -> Rate Limiter1/1, Rate Limiter/1, Switch/2

== system mcb_pmsm_foc_sensorless_CVAC_IF_f28379d/Controller/Subsystem/Inverter ==
  Inverter Signals : Inport
  Code Generation : Subsystem  VariantControl=(codegen)
  Simulation : Subsystem  VariantControl=(sim)
  DutyCycles : Outport  VectorParamsAs1DForOutWhenUnconnected=off

== system mcb_pmsm_foc_sensorless_CVAC_IF_f28379d/Controller/Subsystem/Output Scaling ==
  Vabc_ref : Inport
  En : Inport  Port=2
  Constant : Constant  Value=0.5  OutDataTypeStr=dataType  SampleTime=-1
  Data Type Conversion : DataTypeConversion  OutDataTypeStr=dataType  SaturateOnIntegerOverflow=off  RndMeth=Floor
  One_by_Two : Gain  Gain=0.5  RndMeth=Simplest  OutDataTypeStr=Inherit: Same as input
  Sum : Sum  Inputs=|++
  PWM_Duty_Cycles : Outport
  PWM_Enable : Outport  Port=2
  wires:
  Constant/1 -> Sum/2
  Vabc_ref/1 -> One_by_Two/1
  Sum/1 -> PWM_Duty_Cycles/1  "PWM_Duty_Cycles"
  En/1 -> Data Type Conversion/1
  One_by_Two/1 -> Sum/1
  Data Type Conversion/1 -> PWM_Enable/1

== system mcb_pmsm_foc_sensorless_CVAC_IF_f28379d/Controller/Subsystem1/Calculate Phase Currents ==
  IabOffset : Inport
  Iab_ADC : Inport  Port=2
  Add : Sum  Inputs=-+
  Data Type Conversion : DataTypeConversion  OutDataTypeStr=int32  ConvertRealWorld=Stored Integer (SI)  RndMeth=Simplest  SaturateOnIntegerOverflow=off
  Data_Type : Subsystem  Variant=on
  Inverting / Non-inverting Current measurement amplifier : Gain  Gain=inverter.invertingAmp  RndMeth=Simplest  OutDataTypeStr=Inherit: Same as input
  Iab_meas_PU : Outport  VectorParamsAs1DForOutWhenUnconnected=off
  wires:
  Data Type Conversion/1 -> Add/2
  Add/1 -> Data_Type/1(In1)
  Data_Type/1(Iab_meas_PU) -> Inverting / Non-inverting Current measurement amplifier/1
  Iab_ADC/1 -> Data Type Conversion/1
  Inverting / Non-inverting Current measurement amplifier/1 -> Iab_meas_PU/1
  IabOffset/1 -> Add/1

== system mcb_pmsm_foc_sensorless_CVAC_IF_f28379d/Controller/Subsystem1/HW_Inputs ==
  Sim : Inport
  Sensor Driver Blocks (codegen) : Subsystem  VariantControl=(codegen)
  Sensor Driver Blocks (sim) : Subsystem  VariantControl=(sim)
  Iab_ADC : Outport

== system mcb_pmsm_foc_sensorless_CVAC_IF_f28379d/Inverter and Motor - Plant Model/Simulation/Inverter ==
  Duty_abc : Inport
  Average-Value Inverter : mcbplantlib/Average-Value Inverter
  Constant2 : Constant  Value=inverter.V_dc  OutDataTypeStr=single  SampleTime=-1
  Data Type Conversion1 : DataTypeConversion  OutDataTypeStr=single  RndMeth=Simplest  SaturateOnIntegerOverflow=off
  Rate Transition3 : RateTransition  Deterministic=off  OutPortSampleTime=Ts_inverter
  Vabc : Outport  VectorParamsAs1DForOutWhenUnconnected=off
  wires:
  Data Type Conversion1/1 -> Rate Transition3/1
  Duty_abc/1 -> Data Type Conversion1/1
  Rate Transition3/1 -> Average-Value Inverter/1
  Constant2/1 -> Average-Value Inverter/2
  Average-Value Inverter/1 -> Vabc/1

== system mcb_pmsm_foc_sensorless_CVAC_IF_f28379d/Inverter and Motor - Plant Model/Simulation/Load_Profile (Torque) ==
  Constant : Constant  Value=CVAC_LoadConstant*pmsm.T_rated
  Data Type Conversion : DataTypeConversion  OutDataTypeStr=single  SaturateOnIntegerOverflow=off  RndMeth=Floor
  IIR Filter : mcbcontrolslib/IIR Filter  VariantControl=Low Pass Filter  VariantSelect=Low-pass  FilterConstantInputType=Specify via dialog  Filter_constant=0.0001  InitialOutput=Specify via dialog  InitialOutputValue=0  ExternalReset=none  advancedSettings=off  Ts=50e-6  cutOff_freq=0.31834
  Step : Step  Time=4  SampleTime=Ts_simulink
  Switch : Switch  Criteria=u2 > Threshold  SaturateOnIntegerOverflow=off  InputSameDT=off
  T_load1 : Step  Time=CVAC_LoadStepTime  InitialValue=CVAC_LoadInitial*pmsm.T_rated  FinalValue=CVAC_LoadFinal*pmsm.T_rated  SampleTime=Ts_simulink
  Load_Trq : Outport  VectorParamsAs1DForOutWhenUnconnected=off
  wires:
  T_load1/1 -> Switch/3
  Data Type Conversion/1 -> IIR Filter/1
  IIR Filter/1 -> Load_Trq/1
  Switch/1 -> Data Type Conversion/1
  Step/1 -> Switch/2
  Constant/1 -> Switch/1

== system mcb_pmsm_foc_sensorless_CVAC_IF_f28379d/Inverter and Motor - Plant Model/Simulation/Sensor_Measurements ==
  note: Scaling
  note: Delays
  PhaseCurr : Inport
  Add Offset : Sum  RndMeth=Simplest
  Data Type Conversion4 : DataTypeConversion  OutDataTypeStr=single  RndMeth=Simplest  SaturateOnIntegerOverflow=off
  Delay1 : Delay  DelayLength=PI_params.delay_Currents
  Get ADC Count : Gain  Gain=target.ADC_MaxCount/target.ADC_Vref  OutMin=0  OutMax=target.ADC_MaxCount  OutDataTypeStr=uint16  RndMeth=Simplest
  Get Current Sense Voltage : Gain  Gain=inverter.invertingAmp * inverter.ISenseVoltPerAmp  RndMeth=Simplest  OutDataTypeStr=Inherit: Same as input
  Offset voltage : Gain  Gain=target.ADC_Vref / target.ADC_MaxCount  RndMeth=Simplest
  Saturate at ADC Vref : Saturate  UpperLimit=target.ADC_Vref  LowerLimit=0
  Saturate at inverter Vref : Saturate  UpperLimit=inverter.ISenseVref  LowerLimit=0
  Selector : Selector  InputPortWidth=3  IndexOptions=Index vector (dialog)  Indices=[1 2]  OutputSizes=1
  ~1.65V in ADC counts : Constant  Value=[inverter.CtSensAOffset inverter.CtSensBOffset]  OutDataTypeStr=uint16  SampleTime=-1
  Sim_fb : Outport  VectorParamsAs1DForOutWhenUnconnected=off
  wires:
  Delay1/1 -> Selector/1  "Iab_fb"
  Data Type Conversion4/1 -> Delay1/1
  PhaseCurr/1 -> Data Type Conversion4/1
  Get ADC Count/1 -> Sim_fb/1
  Add Offset/1 -> Saturate at inverter Vref/1
  Saturate at inverter Vref/1 -> Saturate at ADC Vref/1
  ~1.65V in ADC counts/1 -> Offset voltage/1
  Get Current Sense Voltage/1 -> Add Offset/1
  Saturate at ADC Vref/1 -> Get ADC Count/1
  Selector/1 -> Get Current Sense Voltage/1
  Offset voltage/1 -> Add Offset/2

== system mcb_pmsm_foc_sensorless_CVAC_IF_f28379d/Controller/Current Control/Calculate position and speed/Extended EMF Observer ==
  InputSignals : Inport
  En : Inport  Port=2
  Action Port : ActionPort  ActionPortLabel=case [ 1 ]:
  Demux1 : Demux
  Extended EMF Observer : mcbsensorlessestimatorlib/Extended EMF Observer  ParameterBusInput=off  InputUnit=Per-unit  PosOut=Electrical position  BlkSampleTime=Ts  MotorSelection=PMSM  EEMFMultiplier=10  StatorResistance=pmsm.Rs  StatorDaxisInductance=pmsm.Ld  StatorQaxisInductance=pmsm.Lq  MaxApplicationSpeed=pmsm.N_base  PolePairs=pmsm.p  MaxStatorVoltage=PU_System.V_base  MaxStatorCurrent=PU_System.I_base  Alpha=10  EEMFCutoffFreq=EEMFObsCutOffFrq  Kp=250  Ki=200000  N_points=1024  SpeedCutoffFreq=EEMFSpdCutOffFrq  PositionUnit=Per-unit  PositionDataType=dataType  SpeedUnit=Per-unit  PerUnitSpeed=PU_System.N_base  SpeedDataType=dataType  TableDatatype=single
  Logical Operator : Logic  Operator=NOT  IconShape=distinctive  AllPortsSameDT=off  OutDataTypeStr=boolean
  Mux2 : Mux  Inputs=2
  Position/Speed : Outport
  wires:
  Mux2/1 -> Position/Speed/1
  Demux1/3 -> Extended EMF Observer/3  "Ialpha"
  Demux1/4 -> Extended EMF Observer/4  "Ibeta"
  Logical Operator/1 -> Extended EMF Observer/5
  En/1 -> Logical Operator/1
  Demux1/1 -> Extended EMF Observer/1
  Demux1/2 -> Extended EMF Observer/2
  InputSignals/1 -> Demux1/1
  Extended EMF Observer/1 -> Mux2/1
  Extended EMF Observer/2 -> Mux2/2

== system mcb_pmsm_foc_sensorless_CVAC_IF_f28379d/Controller/Current Control/Calculate position and speed/Flux Observer ==
  InputSignals : Inport
  En : Inport  Port=2
  Action Port : ActionPort  ActionPortLabel=case [ 0 ]:
  DC component removal : Subsystem  Commented=through
  Demux1 : Demux
  Flux Observer : mcbpositiondecoderlib/Flux Observer  DataTypeSelect=off  ParameterBusInput=off  MotorSelection=PMSM  BlockInputUnit=Per-unit  PerUnitVoltage=PU_System.V_base  PerUnitCurrent=PU_System.I_base  PositionSelect=on  FluxSelect=off  TorqueSelect=off  PolePairs=4  StatorResistance=pmsm.Rs  StatorDAxisInductance=pmsm.Ld  StatorLeakageInductance=0.0068  RotorLeakageInductance=0.0068  MagnetizingInductance=0.0300  CutoffFreq=3.1863  BlockSampleTime=Ts  PositionUnit=Per-unit  PositionDatatype=dataType  FluxUnit=Weber  PerUnitFlux=0.1  FluxDatatype=single  TorqueUnit=Nm  PerUnitTorque=100  TorqueDatatype=single  DataType=0
  IIR Filter4 : mcbcontrolslib/IIR Filter  VariantControl=Low Pass Filter  VariantSelect=Low-pass  FilterConstantInputType=Specify via dialog  Filter_constant=(2*pi*15*Ts)/(1+(2*pi*15*Ts))  InitialOutput=Specify via dialog  InitialOutputValue=0  ExternalReset=none  advancedSettings=on  Ts=Ts  cutOff_freq=15
  Logical Operator : Logic  Operator=NOT  IconShape=distinctive  AllPortsSameDT=off  OutDataTypeStr=boolean
  Mux2 : Mux  Inputs=2
  Speed Measurement : mcbpositiondecoderlib/Speed Measurement  DiscreteStepInput=off  LastDiscreteStepInput=off  PositionUnit=Per unit  PositionScalingDatatype=uint32  SpeedCalculationMode=Time interval for speed calculation  TempSpeedCalculationMode=Time interval for speed calculation  SampleTimeAsync=Ts  MaximumApplicationSpeed=60000  SpeedResolution=5e-6  DelayLength=10  MaximumMeasurableSpeed=54545.4545  MeasurableSpeedResolution=2.794e-05  SpeedUnit=Per unit based on dialog  TempSpeedUnit=RPM  PerUnitSpeed=PU_System.N_base  SpeedDataType=dataType
  elect2mech : Gain  Gain=1/pmsm.p  RndMeth=Simplest  OutDataTypeStr=Inherit: Same as input
  Position/Speed : Outport
  wires:
  InputSignals/1 -> DC component removal/1(SigIN)
  Mux2/1 -> Position/Speed/1
  Speed Measurement/1 -> IIR Filter4/1
  elect2mech/1 -> Mux2/2
  Demux1/3 -> Flux Observer/3  "Ialpha"
  Demux1/4 -> Flux Observer/4  "Ibeta"
  IIR Filter4/1 -> elect2mech/1
  Logical Operator/1 -> Flux Observer/5
  En/1 -> Logical Operator/1
  Flux Observer/1 -> Mux2/1, Speed Measurement/1
  Demux1/1 -> Flux Observer/1
  Demux1/2 -> Flux Observer/2
  DC component removal/1(SigOUT) -> Demux1/1

== system mcb_pmsm_foc_sensorless_CVAC_IF_f28379d/Controller/Current Control/Closed Loop/Current_Controllers ==
  Id : Inport
  Iq : Inport  Port=2
  Idq_Ref : Inport  Port=3
  DQ Limiter : mcbcontrolslib/DQ Limiter  satMethodInputType=Specify via dialog  satMethodSelected=D-Q equivalence  satLimitInputType=Specify via dialog  Vmax=0.99
  Demux : Demux  Outputs=2
  Mux : Mux
  PI_Controller_Id : Subsystem
  PI_Controller_Iq : Subsystem
  Terminator : Terminator
  Vd_ref : Outport  VectorParamsAs1DForOutWhenUnconnected=off
  Vq_ref : Outport  Port=2  VectorParamsAs1DForOutWhenUnconnected=off
  Idq : Outport  Port=3  VectorParamsAs1DForOutWhenUnconnected=off
  wires:
  Iq/1 -> Mux/4, PI_Controller_Iq/2(I_fb)  "Iq_fb"
  PI_Controller_Id/1(V_ref) -> DQ Limiter/1
  Id/1 -> PI_Controller_Id/2(I_fb), Mux/2  "Id_fb"
  Demux/1 -> PI_Controller_Id/1(I_ref), Mux/1  "Id_Ref"
  Demux/2 -> Mux/3, PI_Controller_Iq/1(I_ref)  "Iq_Ref"
  DQ Limiter/1 -> Vd_ref/1
  DQ Limiter/2 -> Vq_ref/1
  PI_Controller_Iq/1(V_ref) -> DQ Limiter/2
  DQ Limiter/3 -> Terminator/1
  Idq_Ref/1 -> Demux/1
  Mux/1 -> Idq/1

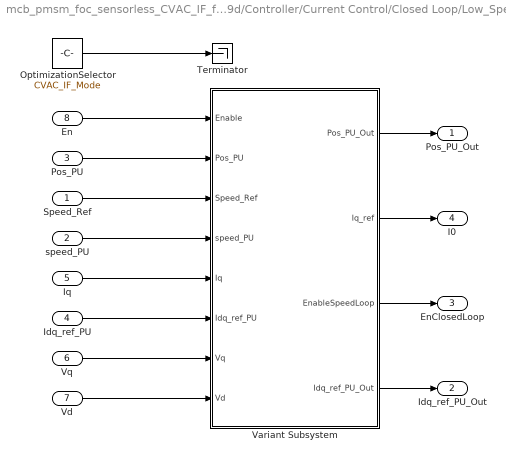
== system mcb_pmsm_foc_sensorless_CVAC_IF_f28379d/Controller/Current Control/Closed Loop/Low_Speed_Control ==
  Speed_Ref : Inport
  speed_PU : Inport  Port=2
  Pos_PU : Inport  Port=3
  Idq_ref_PU : Inport  Port=4
  Iq : Inport  Port=5
  Vq : Inport  Port=6
  Vd : Inport  Port=7
  En : Inport  Port=8
  OptimizationSelector : Constant  Value=CVAC_IF_Mode  OutDataTypeStr=uint32
  Terminator : Terminator
  Variant Subsystem : Subsystem  Variant=on
  Pos_PU_Out : Outport
  Idq_ref_PU_Out : Outport  Port=2
  EnClosedLoop : Outport  Port=3
  I0 : Outport  Port=4
  wires:
  OptimizationSelector/1 -> Terminator/1
  En/1 -> Variant Subsystem/1(Enable)
  speed_PU/1 -> Variant Subsystem/4(speed_PU)
  Idq_ref_PU/1 -> Variant Subsystem/6(Idq_ref_PU)
  Vq/1 -> Variant Subsystem/7(Vq)
  Pos_PU/1 -> Variant Subsystem/2(Pos_PU)
  Speed_Ref/1 -> Variant Subsystem/3(Speed_Ref)
  Iq/1 -> Variant Subsystem/5(Iq)
  Vd/1 -> Variant Subsystem/8(Vd)
  Variant Subsystem/1(Pos_PU_Out) -> Pos_PU_Out/1
  Variant Subsystem/2(Iq_ref) -> I0/1
  Variant Subsystem/3(EnableSpeedLoop) -> EnClosedLoop/1
  Variant Subsystem/4(Idq_ref_PU_Out) -> Idq_ref_PU_Out/1

== system mcb_pmsm_foc_sensorless_CVAC_IF_f28379d/Controller/Hardware Init/Variant Subsystem/Code Generation ==
  note: for BoostXL-DRV8305 connected to LaunchXL-28379D
  note: System Outputs
  note: Enable ADC offset calibration only when motor is not loaded and not rotating due to external factors
  In1 : Inport
  "Calculate ADC Offset " : Subsystem  Priority=1001  TreatAsAtomicUnit=on
  Constant : Constant  Value=inverter.ADCOffsetCalibEnable
  DRV Enable : Subsystem  Priority=1
  Default ADC Offset : Subsystem  Priority=1001  TreatAsAtomicUnit=on
  NOT : Logic  Operator=NOT  IconShape=distinctive  AllPortsSameDT=off  OutDataTypeStr=boolean
  wires:
  In1/1 -> DRV Enable/1(In)
  NOT/1 -> Default ADC Offset/Enable
  Constant/1 -> NOT/1, "Calculate ADC Offset "/Enable

== system mcb_pmsm_foc_sensorless_CVAC_IF_f28379d/Controller/Hardware Init/Variant Subsystem/Simulation ==
  In1 : Inport
  Terminator : Terminator
  wires:
  In1/1 -> Terminator/1

== system mcb_pmsm_foc_sensorless_CVAC_IF_f28379d/Controller/Heartbeat LED/Heartbeat LED/Code generation ==
  In1 : Inport
  Digital Output : c2837xDlib/Digital Output  GPIO_Number=GPIO32~GPIO39  GPIO_Bit0=off  GPIO_BIT0_Toggle=on  GPIO_Bit1=off  GPIO_BIT1_Toggle=off  GPIO_Bit2=on  GPIO_BIT2_Toggle=on  GPIO_Bit3=off  GPIO_BIT3_Toggle=off  GPIO_Bit4=off  GPIO_BIT4_Toggle=off  GPIO_Bit5=off  GPIO_BIT5_Toggle=off  GPIO_Bit6=off  GPIO_BIT6_Toggle=off  GPIO_Bit7=off  GPIO_BIT7_Toggle=off
  wires:
  In1/1 -> Digital Output/1

== system mcb_pmsm_foc_sensorless_CVAC_IF_f28379d/Controller/Heartbeat LED/Heartbeat LED/Simulation ==
  In1 : Inport
  Simulation_Terminator : Terminator
  wires:
  In1/1 -> Simulation_Terminator/1

== system mcb_pmsm_foc_sensorless_CVAC_IF_f28379d/Controller/SCI_Tx/Code Generation/Data_Conditioning_Tx ==
  In1 : Inport
  Data_Type_Fixed_Point : Subsystem  VariantControl=~isequal(dataType,'single')
  Data_Type_Float : Subsystem  VariantControl=isequal(dataType, 'single')
  Data_Log : Outport

== system mcb_pmsm_foc_sensorless_CVAC_IF_f28379d/Controller/SCI_Tx/Code Generation/Data_Logging ==
  note: Fast Serial Data Monitoring (32-bit)
  Data_Log : Inport
  Counter Limited : simulink/Sources/Counter Limited  uplimit=600-1  tsamp=-1
  Data : Subsystem  TreatAsAtomicUnit=on
  End : Subsystem  TreatAsAtomicUnit=on
  If : If  IfExpression=u1 == 0  ElseIfExpressions=u1 == 599
  Merge : Merge  Inputs=3
  Merge1 : Merge  Inputs=3
  Mux : Mux  Inputs=2
  Start : Subsystem  TreatAsAtomicUnit=on
  Width : Width  OutDataTypeMode=All ports same datatype  DataType=uint16
  SCI_Tx : Outport
  wires:
  If/3 -> Data/Action
  Data/1(Data_out) -> Merge/3
  Width/1 -> Data/2(Data_width), Start/2(Data_width), End/2(Data_width)
  Merge/1 -> Mux/1  "SCI_Tx_Data"
  Counter Limited/1 -> If/1
  Start/2(Iteration) -> Merge1/1
  Start/1(Data_out) -> Merge/1
  If/2 -> End/Action
  Merge1/1 -> Mux/2  "SCI_Tx_Iteration"
  If/1 -> Start/Action
  End/1(Data_out) -> Merge/2
  End/2(Iteration) -> Merge1/2
  Data/2(Iteration) -> Merge1/3
  Mux/1 -> SCI_Tx/1
  Data_Log/1 -> Width/1, Start/1(Data), End/1(Data), Data/1(Data)

== system mcb_pmsm_foc_sensorless_CVAC_IF_f28379d/Controller/SCI_Tx/Code Generation/While Iterator Subsystem ==
  Data : Inport
  Iteration : Inport  Port=2
  Add : Sum  Inputs=+-  OutDataTypeStr=Inherit: Same as first input
  Index Vector : MultiPortSwitch  Inputs=1  SaturateOnIntegerOverflow=off  InputSameDT=off
  SCI Transmit : c280xlib/SCI Transmit  sciModule=A  dataHead=''  dataTail=''  frameSize=1  blockingMode=on  outputStatus=off
  While Iterator : WhileIterator  MaxIters=-1  WhileBlockType=do-while  ShowIterationPort=on  OutputDataType=int16
  wires:
  While Iterator/1 -> Add/2, Index Vector/1
  Data/1 -> Index Vector/2
  Index Vector/1 -> SCI Transmit/1
  Add/1 -> While Iterator/1
  Iteration/1 -> Add/1
